simulink library "calculateFeatheredWingAngle"  (R2018a)
settings: Solver=VariableStepAuto  StartTime=0.0  StopTime=10.0  RelTol=1e-3
undefined symbols (not defined in the file): ctrl, plant
libraries: lowLevel x2, controllerComponents x1
settings Model: Creator=mitch  LastModifiedBy=mitch

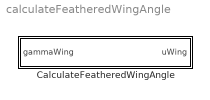
== system calculateFeatheredWingAngle ==
  CalculateFeatheredWingAngle : Subsystem

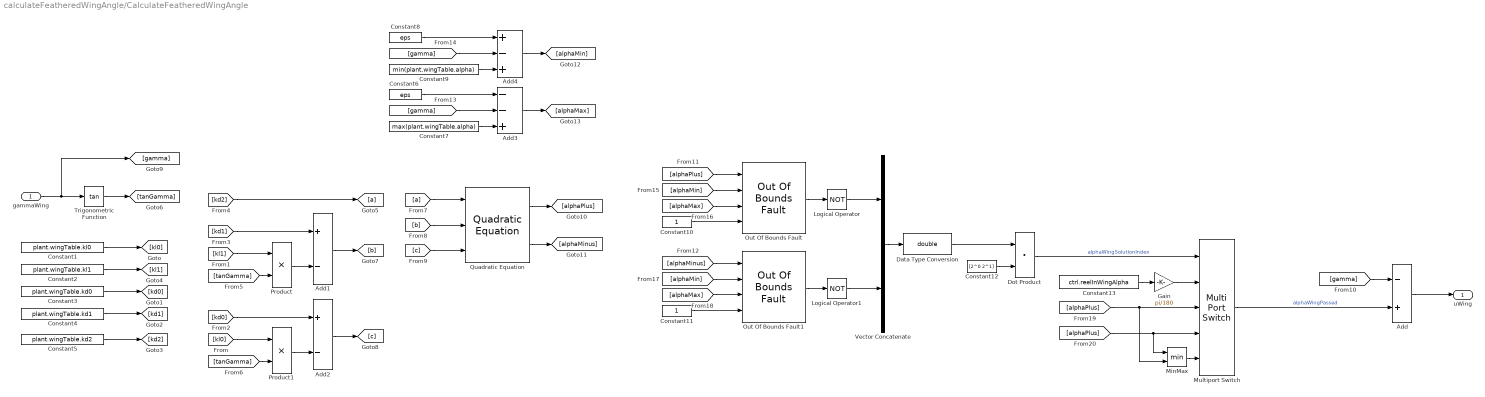
== system calculateFeatheredWingAngle/CalculateFeatheredWingAngle ==
  gammaWing : Inport
  Add : Sum  Inputs=-+
  Add1 : Sum  Inputs=+-
  Add2 : Sum  Inputs=+-
  Add3 : Sum  Inputs=--+
  Add4 : Sum  Inputs=+-+
  Constant1 : Constant  Value=plant.wingTable.kl0
  Constant10 : Constant
  Constant11 : Constant
  Constant12 : Constant  Value=[2^0 2^1]
  Constant13 : Constant  Value=ctrl.reelInWingAlpha
  Constant2 : Constant  Value=plant.wingTable.kl1
  Constant3 : Constant  Value=plant.wingTable.kd0
  Constant4 : Constant  Value=plant.wingTable.kd1
  Constant5 : Constant  Value=plant.wingTable.kd2
  Constant6 : Constant  Value=eps
  Constant7 : Constant  Value=max(plant.wingTable.alpha)
  Constant8 : Constant  Value=eps
  Constant9 : Constant  Value=min(plant.wingTable.alpha)
  Data Type Conversion : DataTypeConversion  OutDataTypeStr=double
  Dot Product : DotProduct  InputSameDT=on  OutDataTypeStr=Inherit: Inherit via internal rule
  Gain : Gain  Gain=pi/180
  Logical Operator : Logic  Operator=NOT  AllPortsSameDT=off  OutDataTypeStr=boolean
  Logical Operator1 : Logic  Operator=NOT  AllPortsSameDT=off  OutDataTypeStr=boolean
  MinMax : MinMax  Inputs=2
  Multiport Switch : MultiPortSwitch  DataPortOrder=Zero-based contiguous  Inputs=4  zeroidx=on
  Out Of Bounds Fault : lowLevel/Out Of Bounds Fault
  Out Of Bounds Fault1 : lowLevel/Out Of Bounds Fault
  Product : Product
  Product1 : Product
  Quadratic Equation : controllerComponents/Quadratic Equation
  Trigonometric Function : Trigonometry  Operator=tan
  Vector Concatenate : Concatenate
  uWing : Outport
  wires:
  Gain/1 -> Multiport Switch/2
  Add/1 -> uWing/1
  Multiport Switch/1 -> Add/2  "alphaWingPassed"
  MinMax/1 -> Multiport Switch/5
  [alphaPlus] -> Multiport Switch/4, MinMax/1
  [alphaPlus] -> Multiport Switch/3, MinMax/2
  Constant13/1 -> Gain/1
  Data Type Conversion/1 -> Dot Product/1
  Dot Product/1 -> Multiport Switch/1  "alphaWingSolutionIndex"
  Constant12/1 -> Dot Product/2
  Vector Concatenate/1 -> Data Type Conversion/1
  Logical Operator1/1 -> Vector Concatenate/2
  Logical Operator/1 -> Vector Concatenate/1
  Out Of Bounds Fault1/1 -> Logical Operator1/1
  Out Of Bounds Fault/1 -> Logical Operator/1
  Constant11/1 -> Out Of Bounds Fault1/4
  [alphaMax] -> Out Of Bounds Fault1/3
  [alphaMin] -> Out Of Bounds Fault1/2
  [alphaMax] -> Out Of Bounds Fault/3
  Constant10/1 -> Out Of Bounds Fault/4
  [alphaMin] -> Out Of Bounds Fault/2
  Add3/1 -> [alphaMax]
  Add4/1 -> [alphaMin]
  [gamma] -> Add4/2
  Constant8/1 -> Add4/1
  Constant9/1 -> Add4/3
  Constant6/1 -> Add3/1
  Constant7/1 -> Add3/3
  [gamma] -> Add3/2
  [alphaMinus] -> Out Of Bounds Fault1/1
  [alphaPlus] -> Out Of Bounds Fault/1
  Quadratic Equation/2 -> [alphaMinus]
  Quadratic Equation/1 -> [alphaPlus]
  [gamma] -> Add/1
  [c] -> Quadratic Equation/3
  [b] -> Quadratic Equation/2
  [a] -> Quadratic Equation/1
  [kl0] -> Product1/1
  [kd0] -> Add2/1
  [tanGamma] -> Product1/2
  Product1/1 -> Add2/2
  Add2/1 -> [c]
  Add1/1 -> [b]
  [kl1] -> Product/1
  [tanGamma] -> Product/2
  Product/1 -> Add1/2
  [kd1] -> Add1/1
  Trigonometric Function/1 -> [tanGamma]
  [kd2] -> [a]
  Constant2/1 -> [kl1]
  Constant3/1 -> [kd0]
  Constant4/1 -> [kd1]
  Constant5/1 -> [kd2]
  Constant1/1 -> [kl0]
  gammaWing/1 -> Trigonometric Function/1, [gamma]
